simulink library "rotateAboutVec"  (R2020a)
settings: Solver=VariableStepAuto  StartTime=0.0  StopTime=10.0  RelTol=1e-3
libraries: xProdMatrix_ul x1
settings Model: Creator=jldanie5  LastModifiedBy=Ayaz
settings DataIOCC: ReturnWorkspaceOutputs=off
settings DebuggingCC: ArithmeticOperatorsInVariantConditions=warning
settings SFSimCC: CustomCodeUndefinedFunction=UseInterfaceOnly

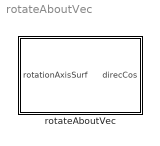
== system rotateAboutVec ==
  rotateAboutVec : Subsystem  mask{ang=0}
      mask prompts: ang "Angle to rotate in degrees (right hand rule)"

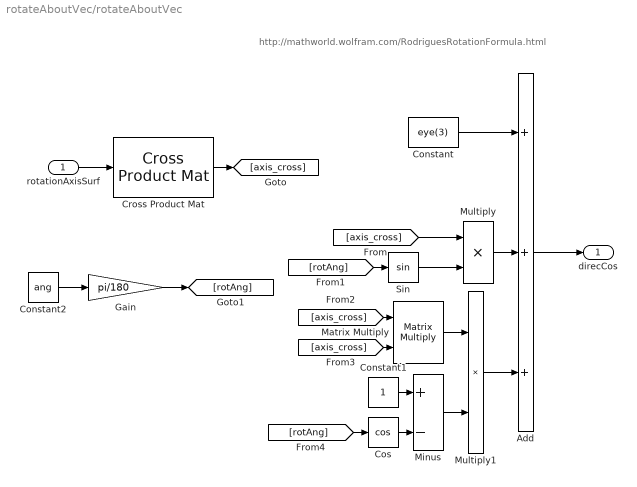
== system rotateAboutVec/rotateAboutVec ==
  note: http://mathworld.wolfram.com/RodriguesRotationFormula.html
  rotationAxisSurf : Inport
  Add : Sum  Inputs=+++
  Constant : Constant  Value=eye(3)  VectorParams1D=off
  Constant1 : Constant
  Constant2 : Constant  Value=ang
  Cos : Trigonometry  Operator=cos
  Cross Product Mat : xProdMatrix_ul/Cross Product Mat  SystemSampleTime=-1  Latency=0  AutoFrameSizeCalculation=off
  Gain : Gain  Gain=pi/180
  Matrix Multiply : Product  Multiplication=Matrix(*)
  Minus : Sum  Inputs=+-
  Multiply : Product
  Multiply1 : Product
  Sin : Trigonometry
  direcCos : Outport  VectorParamsAs1DForOutWhenUnconnected=off
  wires:
  rotationAxisSurf/1 -> Cross Product Mat/1
  Cross Product Mat/1 -> [axis_cross]
  Constant/1 -> Add/1
  [axis_cross] -> Multiply/1
  Constant2/1 -> Gain/1
  [rotAng] -> Sin/1
  Sin/1 -> Multiply/2
  Multiply/1 -> Add/2
  Matrix Multiply/1 -> Multiply1/1
  [axis_cross] -> Matrix Multiply/1
  [axis_cross] -> Matrix Multiply/2
  Minus/1 -> Multiply1/2
  [rotAng] -> Cos/1
  Cos/1 -> Minus/2
  Constant1/1 -> Minus/1
  Multiply1/1 -> Add/3
  Add/1 -> direcCos/1
  Gain/1 -> [rotAng]
